simulink model "Problem_4"  (R2020a)
settings: Solver=VariableStepAuto  StartTime=0.0  StopTime=10.0  RelTol=1e-3
model workspace (MAT data in the model file):
  x = Simulink.Parameter
  x.Value = 1
  x.DataType = 'auto'
  x.Dimensions = [1 1]
settings Model: Creator=hp  LastModifiedBy=hp

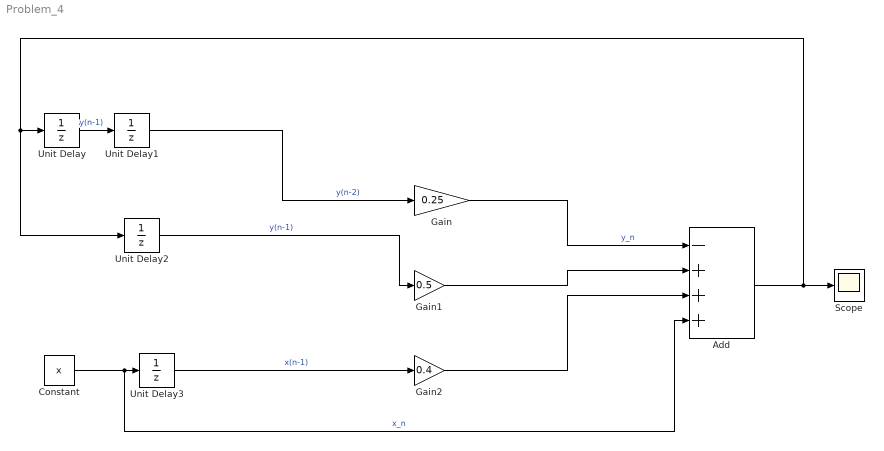
== system Problem_4 ==
  Add : Sum  Inputs=-+++
  Constant : Constant  Value=x
  Gain : Gain  Gain=0.25
  Gain1 : Gain  Gain=0.5
  Gain2 : Gain  Gain=0.4
  Scope : Scope
  Unit Delay{,1..3} (4 alike) : UnitDelay  SampleTime=-1  HasFrameUpgradeWarning=on
  wires:
  Add/1 -> Unit Delay2/1, Unit Delay/1, Scope/1
  Gain1/1 -> Add/2
  Gain2/1 -> Add/3
  Gain/1 -> Add/1  "y_n"
  Unit Delay2/1 -> Gain1/1  "y(n-1)"
  Unit Delay3/1 -> Gain2/1  "x(n-1)"
  Constant/1 -> Unit Delay3/1, Add/4  "x_n"
  Unit Delay/1 -> Unit Delay1/1  "y(n-1)"
  Unit Delay1/1 -> Gain/1  "y(n-2)"
